simulink model "current_control_ver15a"  (R2015a)
settings: Solver=ode23t  StartTime=0.0  StopTime=1  MaxStep=1e-4  RelTol=1e-5  AbsTol=1e-4
undefined symbols (not defined in the file): j, P
libraries: fl_lib x9, nesl_utility x9, pe_lib x3, ThreePhaseExamples_lib x1
Description:
  | Three-Phase Custom PMSM
  | 
  | This example shows a custom Simscape(TM) implementation of
  | a Permanent Magnet Synchronous Machine (PMSM). To view the
  | PMSM source code, double-click on the motor block and then
  | click on the hyperlink 'Source code'. This test circuit shows the
  | PMSM being used as a generator, the rectifier block converting
  | the induced AC back EMFs to a DC voltage which is in turn
  | applied to a resistive load.
  | 
  | 
  | 
  | Copyright 2008-2016 The MathWorks, Inc.
settings Model: CovSFcnEnable=off  Creator=MathWorks  LastModifiedBy=hbjo
settings DebuggingCC: UnderspecifiedInitializationDetection=Classic  MergeDetectMultiDrivingBlocksExec=none
settings SimscapeCC: SimscapeLogDataHistory=50000
settings ConfigurationSet: Description=Simscape Multibody

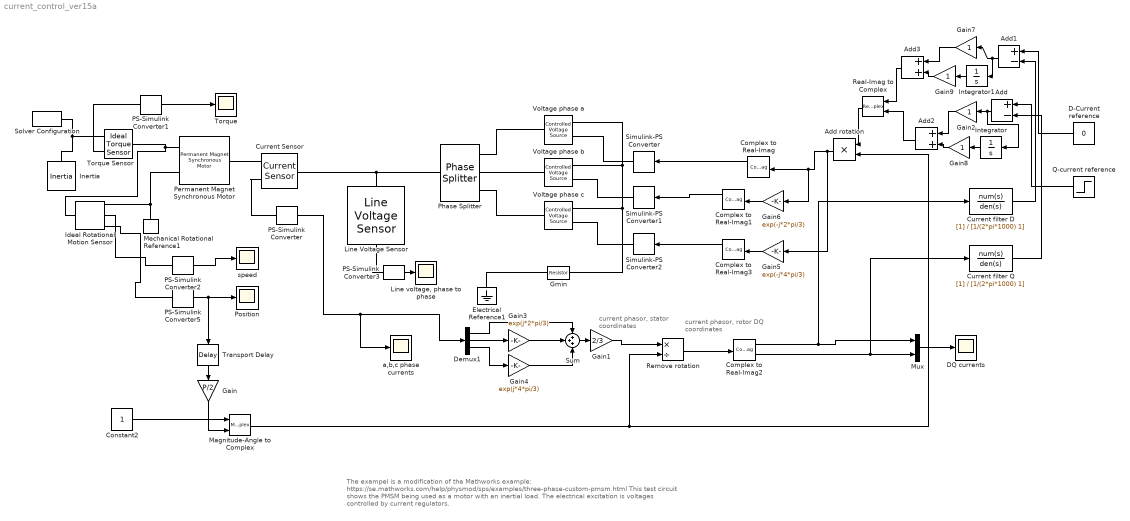
== system current_control_ver15a ==
  note: current phasor,
      |  stator coordinates
  note: current phasor,
      | rotor DQ coordinates
  note: The exampel is a modification of the Mathworks example: https://se.mathworks.com/help/physmod/sps/examples/three-phase-custom-pmsm.html
      | This test circuit shows the PMSM being used as a motor with an inertial load.
      | The electrical excitation is voltages controlled by current regulators.
  Add : Sum  Inputs=+-
  Add rotation : Product
  Add1 : Sum  Inputs=+-
  Add2 : Sum
  Add3 : Sum
  Complex to Real-Imag{,1..3} (4 alike) : ComplexToRealImag
  Constant2 : Constant
  Current Sensor : pe_lib/Sensors/Current Sensor
  Current filter D : TransferFcn  Denominator=[1/(2*pi*1000) 1]
  Current filter Q : TransferFcn  Denominator=[1/(2*pi*1000) 1]
  D-Current reference : Constant  Value=0
  DQ currents : Scope
      settings: TimeRange=1  LimitDataPoints=on  MaxDataPoints=50000  SaveToWorkspace=off  YMin=-0.16198  YMax=12.49459  SampleTime=-1  Decimation=10
  Demux1 : Demux  Outputs=3
  Electrical Reference1 : fl_lib/Electrical/Electrical Elements/Electrical Reference
  Gain : Gain  Gain=P/2
  Gain1 : Gain  Gain=2/3
  Gain{2,7..9} (4 alike) : Gain  SaturateOnIntegerOverflow=on  OutDataTypeStr=Inherit: Same as input  ParamDataTypeStr=Inherit: Same as input
  Gain3 : Gain  Gain=exp(j*2*pi/3)
  Gain4 : Gain  Gain=exp(j*4*pi/3)
  Gain5 : Gain  Gain=exp(-j*4*pi/3)
  Gain6 : Gain  Gain=exp(-j*2*pi/3)
  Gmin : fl_lib/Electrical/Electrical Elements/Resistor  R=1e9 Ohm  i_specify=off  i_priority=High  i=0 A  v_specify=off  v_priority=High  v=0 V
  Ideal Rotational Motion Sensor : fl_lib/Mechanical/Mechanical Sensors/Ideal Rotational Motion Sensor  offset=0 rad
  Inertia : fl_lib/Mechanical/Rotational Elements/Inertia  inertia=J kg*m^2  w_specify=off  w_priority=High  w=0 rad/s  t_specify=off  t_priority=None  t=0 N*m
  Integrator : Integrator
  Integrator1 : Integrator
  Line Voltage Sensor : pe_lib/Sensors/Line Voltage Sensor
  "Line voltage, phase to phase" : Scope
      settings: TimeRange=auto  LimitDataPoints=on  MaxDataPoints=50000  SaveToWorkspace=off  SaveName=ScopeData3  YMin=-119.07849  YMax=205.68103  SampleTime=-1  Decimation=10
  Magnitude-Angle to Complex : MagnitudeAngleToComplex
  Mechanical Rotational Reference1 : fl_lib/Mechanical/Rotational Elements/Mechanical Rotational Reference
  Mux : Mux  Inputs=2
  PS-Simulink Converter{,1..3,5} (5 alike) : nesl_utility/PS-Simulink Converter  PhysicalDomain=network_engine_domain  SubClassName=ps_output  LeftPortType=input  RightPortType=output  PseudoPeriodic=off  Frequencies=[]  AffineConversion=off
  Permanent Magnet Synchronous Motor : ThreePhaseExamples_lib/Permanent Magnet Synchronous Motor  nPolePairs=P/2  pm_flux_linkage=psi Wb  Ld=L H  Lq=L H  Rs=R Ohm  wNominal=0 rad/s  angular_position_diff_specify=off  angular_position_diff_priority=None  angular_position_diff=0 rad  i_d_specify=off  i_d_priority=High  i_d=0 A  i_q_specify=off  i_q_priority=High  i_q=0 A
  Phase Splitter : pe_lib/Connections/Phase Splitter
  Position : Scope
      settings: TimeRange=1  LimitDataPoints=on  MaxDataPoints=50000  SaveToWorkspace=off  SaveName=ScopeData2  YMin=-44.40189  YMax=1374.23605  SampleTime=-1  Decimation=10
  Q-current reference : Step  Time=0.1  After=10  SampleTime=0
  Real-Imag to Complex : RealImagToComplex
  Remove rotation : Product  Inputs=*/
  Simulink-PS Converter : nesl_utility/Simulink-PS Converter  PhysicalDomain=network_engine_domain  SubClassName=ps_input  LeftPortType=input  RightPortType=output  PseudoPeriodic=off  Frequencies=[]  NoiseDistribution=none  NoiseParameters=[]  AffineConversion=off  InputFiltering=off  SimscapeFilterOrder=1  InputFilterTimeConstant=0.001  UdotUserProvided=1
  Simulink-PS Converter1 : nesl_utility/Simulink-PS Converter  PhysicalDomain=network_engine_domain  SubClassName=ps_input  LeftPortType=input  RightPortType=output  PseudoPeriodic=off  Frequencies=[]  NoiseDistribution=none  NoiseParameters=[]  AffineConversion=off  InputFiltering=off  SimscapeFilterOrder=1  InputFilterTimeConstant=0.001  UdotUserProvided=1
  Simulink-PS Converter2 : nesl_utility/Simulink-PS Converter  PhysicalDomain=network_engine_domain  SubClassName=ps_input  LeftPortType=input  RightPortType=output  PseudoPeriodic=off  Frequencies=[]  NoiseDistribution=none  NoiseParameters=[]  AffineConversion=off  InputFiltering=off  SimscapeFilterOrder=1  InputFilterTimeConstant=0.001  UdotUserProvided=1
  Solver Configuration : nesl_utility/Solver Configuration  PhysicalDomain=network_engine_domain  SubClassName=solver  LeftPortType=input  RightPortType=generic  Accelerate=off  Tones=[]  Harmonics=[]  SimulateNoise=off  Profile=off  UseLocalSampling=off  EnableSwitchedLinearOptims=on  FrequencyDomain=off  UseCCode=off  RelTol=0.001  AbsTol=1e-06  MinStep=1e-09  ToWorkspace=off  RevertToSquareIcSolve=off  NumHomotopyIterations=100  PhasorMode=off  PhasorModeNumHarmonics=1  OverrideAbsTol=off  DoDC=off  ResidualTolerance=1e-9  UseLocalSolver=on  LocalSolverChoice=NE_BACKWARD_EULER_ADVANCER  LocalSolverSampleTime=1e-5  DoFixedCost=on  MaxNonlinIter=3  MaxModeIter=2  LinearAlgebra=Sparse  DelaysMemoryBudget=1024  AutomaticFiltering=on  FilteringTimeConstant=0.001
  Sum : Sum  Inputs=+++
  Torque : Scope
      settings: TimeRange=1  LimitDataPoints=on  MaxDataPoints=50000  SaveToWorkspace=off  SaveName=ScopeData7  YMin=-662.90841  YMax=575.45604  SampleTime=-1  Decimation=10
  Torque Sensor : fl_lib/Mechanical/Mechanical Sensors/Ideal Torque Sensor
  Transport Delay : TransportDelay  DelayTime=1e-5
  Voltage phase a : fl_lib/Electrical/Electrical Sources/Controlled Voltage Source
  Voltage phase b : fl_lib/Electrical/Electrical Sources/Controlled Voltage Source
  Voltage phase c : fl_lib/Electrical/Electrical Sources/Controlled Voltage Source
  a,b,c phase currents : Scope
      settings: TimeRange=1  LimitDataPoints=on  MaxDataPoints=50000  SaveToWorkspace=off  SaveName=ScopeData2  YMin=-16.94157  YMax=16.5164  SampleTime=-1  Decimation=10
  speed : Scope
      settings: TimeRange=1  LimitDataPoints=on  MaxDataPoints=50000  SaveToWorkspace=off  YMin=-82.37239  YMax=1266.31166  SampleTime=-1  Decimation=10
  wires:
  PS-Simulink Converter1/1 -> Torque/1
  PS-Simulink Converter3/1 -> "Line voltage, phase to phase"/1
  PS-Simulink Converter2/1 -> speed/1
  PS-Simulink Converter5/1 -> Transport Delay/1, Position/1
  Complex to Real-Imag1/1 -> Simulink-PS Converter1/1
  Complex to Real-Imag/1 -> Simulink-PS Converter/1
  Gain6/1 -> Complex to Real-Imag1/1
  Constant2/1 -> Magnitude-Angle to Complex/1
  Transport Delay/1 -> Gain/1
  Gain/1 -> Magnitude-Angle to Complex/2
  Magnitude-Angle to Complex/1 -> Add rotation/2, Remove rotation/2
  Demux1/2 -> Gain3/1
  Demux1/3 -> Gain4/1
  Gain3/1 -> Sum/2
  Demux1/1 -> Sum/1
  Gain4/1 -> Sum/3
  Mux/1 -> DQ currents/1
  Complex to Real-Imag2/1 -> Current filter D/1, Mux/1
  Complex to Real-Imag2/2 -> Current filter Q/1, Mux/2
  Sum/1 -> Gain1/1
  Gain1/1 -> Remove rotation/1
  Q-current reference/1 -> Add/1
  Remove rotation/1 -> Complex to Real-Imag2/1
  Gain5/1 -> Complex to Real-Imag3/1
  Complex to Real-Imag3/1 -> Simulink-PS Converter2/1
  PS-Simulink Converter/1 -> Demux1/1, a,b,c phase currents/1
  Add/1 -> Integrator/1, Gain2/1
  Real-Imag to Complex/1 -> Add rotation/1
  Add rotation/1 -> Gain5/1, Gain6/1, Complex to Real-Imag/1
  Current filter Q/1 -> Add/2
  D-Current reference/1 -> Add1/1
  Add1/1 -> Integrator1/1, Gain7/1
  Current filter D/1 -> Add1/2
  Gain2/1 -> Add2/1
  Integrator/1 -> Gain8/1
  Gain8/1 -> Add2/2
  Add2/1 -> Real-Imag to Complex/2
  Integrator1/1 -> Gain9/1
  Gain9/1 -> Add3/2
  Gain7/1 -> Add3/1
  Add3/1 -> Real-Imag to Complex/1
  connections:
  Permanent Magnet Synchronous Motor/RConn2 -- Ideal Rotational Motion Sensor/RConn1 -- Mechanical Rotational Reference1/LConn1
  Current Sensor/RConn1 -- PS-Simulink Converter/LConn1
  Ideal Rotational Motion Sensor/LConn1 -- Torque Sensor/LConn1 -- Permanent Magnet Synchronous Motor/RConn1
  Inertia/LConn1 -- Torque Sensor/RConn1 -- Solver Configuration/RConn1
  Electrical Reference1/LConn1 -- Gmin/LConn1
  PS-Simulink Converter3/LConn1 -- Line Voltage Sensor/RConn1
  Torque Sensor/RConn2 -- PS-Simulink Converter1/LConn1
  Phase Splitter/LConn1 -- Line Voltage Sensor/LConn1 -- Current Sensor/LConn1
  Phase Splitter/RConn1 -- Voltage phase a/LConn1
  Phase Splitter/RConn2 -- Voltage phase b/LConn1
  Voltage phase b/RConn2 -- Gmin/RConn1 -- Voltage phase c/RConn2 -- Voltage phase a/RConn2
  PS-Simulink Converter2/LConn1 -- Ideal Rotational Motion Sensor/RConn2
  PS-Simulink Converter5/LConn1 -- Ideal Rotational Motion Sensor/RConn3
  Voltage phase a/RConn1 -- Simulink-PS Converter/RConn1
  Voltage phase b/RConn1 -- Simulink-PS Converter1/RConn1
  Voltage phase c/LConn1 -- Phase Splitter/RConn3
  Simulink-PS Converter2/RConn1 -- Voltage phase c/RConn1
  Permanent Magnet Synchronous Motor/LConn1 -- Current Sensor/RConn2
